simulink model "FirstPrincValveOnly_Testing"  (R2025b)
settings: Solver=VariableStepAuto  StartTime=0.0  StopTime=10.0  RelTol=1e-3
undefined symbols (not defined in the file): CdA_table, epsilon, P_1_ox, psi_to_Pa, rho_ox, theta_bp
settings Model: Creator=gruby  LastModifiedBy=gruby

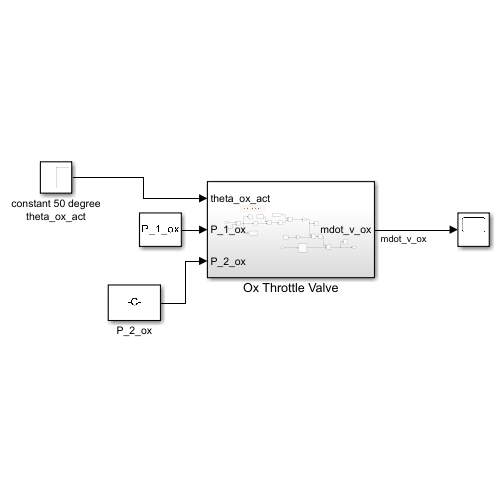
[thumbnail: Simulink's stored preview of the top-level diagram]
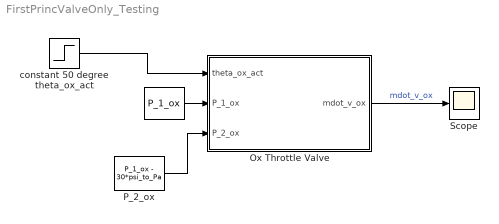
== system FirstPrincValveOnly_Testing ==
  " " : Constant  Value=P_1_ox
  Ox Throttle Valve : Subsystem
  P_2_ox : Constant  Value=P_1_ox - 30*psi_to_Pa
  Scope : Scope
      settings: ActiveDisplayYMinimum=0.041576725328028336  ActiveDisplayYMaximum=0.24157672532802835
  constant 50 degree theta_ox_act : Step  Time=10  Before=50  After=50  SampleTime=0
  wires:
  " "/1 -> Ox Throttle Valve/2(P_1_ox)
  P_2_ox/1 -> Ox Throttle Valve/3(P_2_ox)
  constant 50 degree theta_ox_act/1 -> Ox Throttle Valve/1(theta_ox_act)
  Ox Throttle Valve/1(mdot_v_ox) -> Scope/1  "mdot_v_ox"

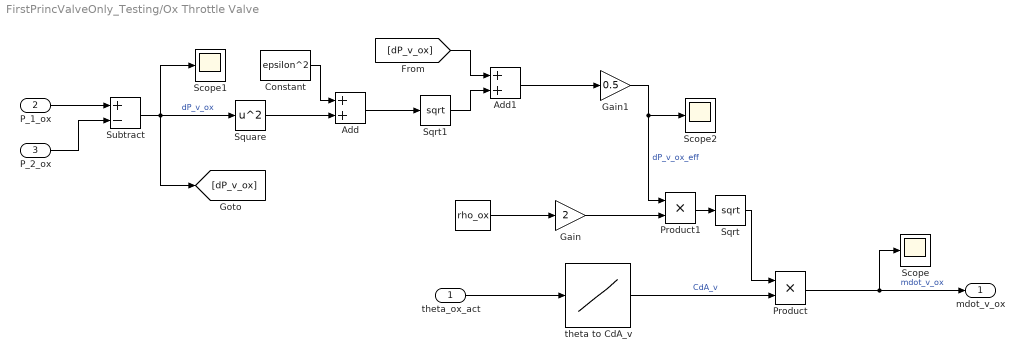
== system FirstPrincValveOnly_Testing/Ox Throttle Valve ==
  theta_ox_act : Inport
  P_1_ox : Inport  Port=2
  P_2_ox : Inport  Port=3
  "  " : Constant  Value=rho_ox
  Add : Sum
  Add1 : Sum
  Constant : Constant  Value=epsilon^2
  Gain : Gain  Gain=2
  Gain1 : Gain  Gain=0.5
  Product : Product
  Product1 : Product
  Scope : Scope
      settings: ActiveDisplayYMinimum=-1  ActiveDisplayYMaximum=1  DataLoggingVariableName=ScopeData6
  Scope1 : Scope
      settings: ActiveDisplayYMinimum=-1  ActiveDisplayYMaximum=1  DataLoggingVariableName=ScopeData10
  Scope2 : Scope
      settings: ActiveDisplayYMinimum=-1  ActiveDisplayYMaximum=1  DataLoggingVariableName=ScopeData19
  Sqrt : Sqrt
  Sqrt1 : Sqrt
  Square : Math  Operator=square
  Subtract : Sum  Inputs=+-
  theta to CdA_v : Lookup_n-D  NumberOfTableDimensions=1  BreakpointsForDimension1=theta_bp  Table=CdA_table  ExtrapMethod=Clip  UseLastTableValue=on  InternalRulePriority=Speed  RndMeth=Simplest
  mdot_v_ox : Outport
  wires:
  Subtract/1 -> [dP_v_ox], Square/1, Scope1/1  "dP_v_ox"
  Sqrt/1 -> Product/1
  "  "/1 -> Gain/1
  Product/1 -> Scope/1, mdot_v_ox/1  "mdot_v_ox"
  Gain/1 -> Product1/2
  theta to CdA_v/1 -> Product/2  "CdA_v"
  Product1/1 -> Sqrt/1
  theta_ox_act/1 -> theta to CdA_v/1
  P_1_ox/1 -> Subtract/1
  P_2_ox/1 -> Subtract/2
  Square/1 -> Add/2
  Constant/1 -> Add/1
  Add/1 -> Sqrt1/1
  [dP_v_ox] -> Add1/1
  Sqrt1/1 -> Add1/2
  Add1/1 -> Gain1/1
  Gain1/1 -> Product1/1, Scope2/1  "dP_v_ox_eff"
